simulink model "test_nn"  (R2020b)
settings: Solver=VariableStepAuto  StartTime=0.0  StopTime=200  RelTol=1e-3
undefined symbols (not defined in the file or in its folder): w
libraries: fuzblock x1, powerlib x1
settings Model: SimulationMode=accelerator  Creator=maloc  LastModifiedBy=maloc
settings SFSimCC: SimTargetLang=C++

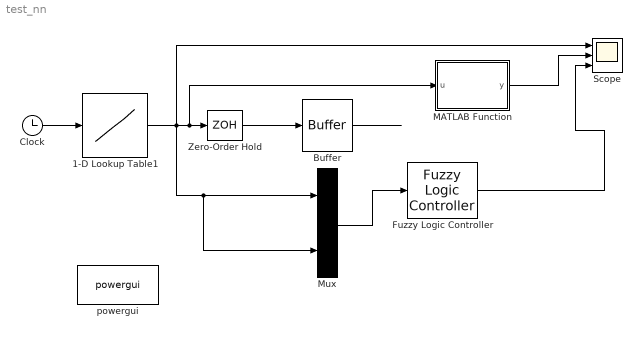
== system test_nn ==
  1-D Lookup Table1 : Lookup_n-D  NumberOfTableDimensions=1  BreakpointsForDimension1=t  Table=w  InternalRulePriority=Speed  RndMeth=Simplest  InputSameDT=on
  Buffer : Buffer  N=1000  OutputFrames=off
  Clock : Clock
  Fuzzy Logic Controller : fuzblock/Fuzzy Logic  Controller  FIS=fuzzy_test  OutputSampleNumber=10  DataType=double  FuzzifiedInputs=off  RuleFiringStrengths=off  RuleOutputs=off  AggregatedOutputs=off  SimulateUsing=Code generation  OutOfRangeInputValueMessage=warning  NoRuleFiredMessage=warning  EmptyOutputFuzzySetMessage=warning
  MATLAB Function : MATLAB Function  TreatAsAtomicUnit=on
  Mux : Mux  Inputs=2
  Scope : Scope  NumInputPorts=3
  Zero-Order Hold : ZeroOrderHold  SampleTime=1e-4
  powergui : powerlib/powergui  Priority=1  SimulationMode=Discrete  SampleTime=1e-4  frequency=60  Iterations=50  frequencyindice=60  Pbase=100e6  ErrMax=1e-4  UnitsV=kV  UnitsW=MW  buscounter=0  FunctionMessages=off  echomessages=off  EnableUseOfTLC=off  CurrentSourceSwitches=off  DisableSnubberDevices=off  DisableRonSwitches=off  DisableVfSwitches=off  DisplayEquations=off  AutomaticDiscreteSolvers=off  SolverType=Tustin/Backward Euler (TBE)  Interpol=off  ExternalGateDelay=off  methode=off  Ts=100  x0status=blocks  SPID=on  SwTol=0  HookPort=off  NonlinearTolerance=1e-4  nMaxIteration=100  ContinueOnMaxIteration=off  RestoreLinks=warning  ResistiveCurrentMeasurement=off  Frange=[0:2:500]  Ylog=off  Xlog=on  ShowGrid=off  save=off  variable=ZData  structure=0  ZoomFFT=off  StartTime=0.0  cycles=1  DisplayStyle=1  fundamental=60  FreqAxis=off  MaxFrequency=1000  frequencyindicesteady=1  RmsSteady=1  display=off
  wires:
  1-D Lookup Table1/1 -> Mux/2, Mux/1, Scope/1, MATLAB Function/1(u), Zero-Order Hold/1
  Buffer/1 -> ?
  Clock/1 -> 1-D Lookup Table1/1
  Zero-Order Hold/1 -> Buffer/1
  MATLAB Function/1(y) -> Scope/2
  Fuzzy Logic Controller/1 -> Scope/3
  Mux/1 -> Fuzzy Logic Controller/1

== matlab function test_nn/MATLAB Function ==
  settings: updateMethod=DISCRETE  sampleTime=1e-4
  data: u input; y output
function y = fcn(u)
% persistent mynet;
% 
% if isempty(mynet)
%     mynet = coder.loadDeepLearningNetwork('net_to_test.mat');
% end
% m = classify(mynet, u');
% if m(end) == 'takeoff'
%     y = 0;
% elseif m(end) == 'climb'
%     y=1;
% elseif m(end) == 'cruise'
%     y=2;
% elseif m(end) == 'descend'
%     y=3;
% end

% persistent myfis;
% 
% if isempty(myfis)
%     myfis = getFISCodeGenerationData('best_sol.fis');
% end
% 
% m = evalfis(myfis,[0.5 0.5]);
% y = m(1);

y = 1;
